simulink model "c6711dskafxr"  (Simulink 6.0)
settings: Solver=FixedStepDiscrete  SolverMode=SingleTasking  StartTime=0.0  StopTime=inf  RelTol=1e-3  AbsTol=1e-6
PreLoadFcn:
  | load dspafxr;
libraries: c6711dsklib x3, c6000tgtpreflib x1, dspsigops x1
settings Model: RequirementInfo=9  Creator=don  LastModifiedBy=thartley  ExtModeTrigMode=oneshot  ExtModeArmWhenConnect=off  ProdHWDeviceType=TI C6000
settings DataIOCC: LimitDataPoints=off  SaveOutput=off  SaveTime=off  SignalLoggingName=sigsOut
settings OptimizationCC: BlockReduction=off  BooleanDataType=off  InlineInvariantSignals=off  RollThreshold=2
settings DebuggingCC: CheckExecutionContextPreStartOutputMsg=on  CheckExecutionContextRuntimeOutputMsg=on  SolverPrmCheckMsg=none  IntegerOverflowMsg=none
settings HardwareCC: ProdBitPerLong=40  ProdEndianess=LittleEndian  ProdHWDeviceType=TI C6000
settings ModelReferenceCC: UpdateModelReferenceTargets=IfOutOfDate
settings RTWCC: SystemTargetFile=ti_c6000.tlc  TemplateMakefile=ti_c6000.tmf  ProcessScript=ti_c6000_make_rtw_hook
settings CodeAppCC: PrefixModelToSubsysFcnNames=off
settings STFCustomTargetCC: TargetFcnLib=ansi_tfl_tmw.mat  MatFileLogging=on  LifeSpan=inf  SystemTargetFile=ti_c6000.tlc  ActivateCallback=c6000_callback('ActivateCallback',hSrc,hDlg);
settings GRTTargetCC: ModelReferenceCompliant=off  LifeSpan=inf
settings CustomProperty: DataType=RTWOptions_EnumType_S__A_matlab_toolbox_rtw_targets_tic6000_tic6000_ti_c6000_BoardType  Value=C6711DSK
settings EnumStrPairs: String=C6416DSK
settings SFSimCC: SFSimApplyToAllLibs=on  SFSimBuildMode=Incremental

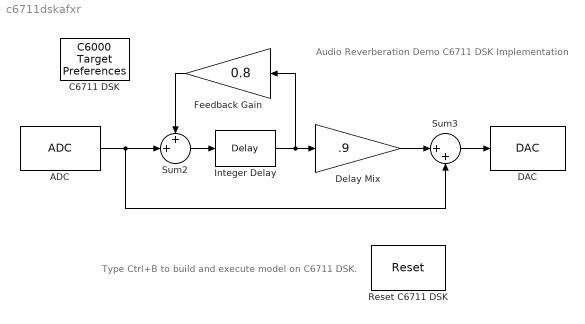
== system c6711dskafxr ==
  note: Type Ctrl+B to build
      | and execute model
      | on C6711 DSK.
  note: Audio Reverberation Demo
      | C6711 DSK Implementation
  ADC : c6711dsklib/ADC  ADCsource=Mic In  MicGain=on  OutputDataType=Double  Scaling=Normalize  SourceGain=0.0  FrameSize=64
  C6711 DSK : c6000tgtpreflib/C6000 Target Preferences
  DAC : c6711dsklib/DAC  Scaling=Normalize  DacAtten=0.0  OverflowMode=Saturate
  Delay Mix : Gain  Gain=.9  SaturateOnIntegerOverflow=on
  Feedback Gain : Gain  Orientation=left  Gain=0.8  SaturateOnIntegerOverflow=on
  Integer Delay : dspsigops/Delay  dly_unit=Samples  delay=1800  ic_detail=off  dif_ic_for_ch=off  dif_ic_for_dly=off  ic=0  reset_popup=None
  Reset C6711 DSK : c6711dsklib/Reset
  Sum2 : Sum  Inputs=++|  SaturateOnIntegerOverflow=on  InputSameDT=on
  Sum3 : Sum  Inputs=|++  SaturateOnIntegerOverflow=on  InputSameDT=on
  wires:
  Sum3/1 -> DAC/1
  ADC/1 -> Sum2/2, Sum3/2
  Sum2/1 -> Integer Delay/1
  Feedback Gain/1 -> Sum2/1
  Integer Delay/1 -> Delay Mix/1, Feedback Gain/1
  Delay Mix/1 -> Sum3/1
